simulink model "hostComms_backup_twoLoops"  (R2014b)
settings: Solver=FixedStepDiscrete  StartTime=0.0  StopTime=inf  RelTol=1e-3
InitFcn:
  | initCV;
  | 
  | fprintf('NXT init\n');
  | 
  | %try
  |  n = comms.Bt(RobotID.NXT);
  |  n.reset();
  |  n.init();
  | fprintf('NXT init done\n');
StopFcn:
  | %figure;
  | %plot(SpheroPos.signals.values(:,1), SpheroPos.signals.values(:, 2), 'kx');
  | %hold on;
  | %plot(points(:, 1), points(:, 2), 'ro');
  | %hold off
  | %axis([0 640 0 480])
  | 
  | %distEnd =  pdist([points(end, :); SpheroPos.signals.values(end, :)])
undefined symbols (not defined in the file or in its folder): angleBlue, angleOrange, curPos, curPosBlue, curPosOrange, desPos, desPosBlue, desPosOrange, Done, DoneBlue, DoneOrange, dThresh, hardcodeAngle, IsPositionTracked, IsSkeletonTracked, JointDepthIndices, JointImageIndices, JointTrackingState, JointWorldCoordinates, none, PositionDepthIndices, PositionImageIndices, PositionWorldCoordinates, posVectBlue, posVectOrange, SegmentationData, SkeletonTrackingID, Stateflow, tClose, tOpen, tSpheroStop, velocity, velocityBlue, velocityOrange, videoinput, z1Speed, z2Speed, zumoInitCentroids
undefined symbols (not defined in the file): Kd, Ki, Kp, restartspeed, RobotID, stopRadius, stopspeed
libraries: hostCommsLib x3, minionLogic x3, visiontextngfix x2, visionsinks x2, simulink x1, imaqlib x1, aerolibanimutils x1, dspvision x1
settings Model: DataDictionary=hostData.sldd  Creator=scastro  LastModifiedBy=gsalhotr

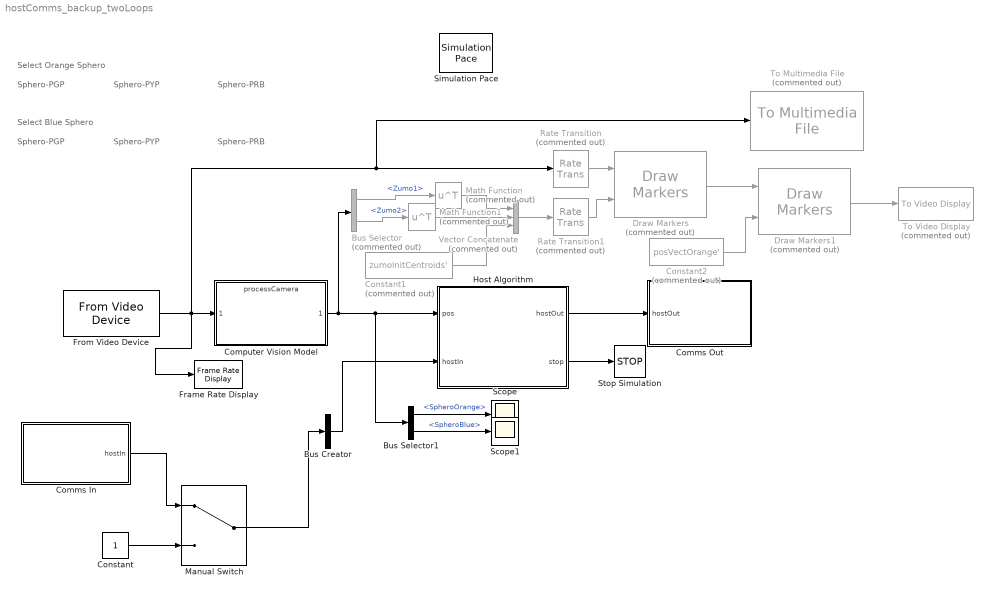
== system hostComms_backup_twoLoops ==
  note: Select Orange Sphero
  note: Sphero-PGP
  note: Sphero-PYP
  note: Sphero-PRB
  note: Select Blue Sphero
  note: Sphero-PGP
  note: Sphero-PYP
  note: Sphero-PRB
  Bus Creator : BusCreator  Inputs=1  OutDataTypeStr=Bus: CommsIn
  Bus Selector : BusSelector  Commented=on  DialogController=Simulink.DDGSource_BusSelector  OutputSignals=Zumo1,Zumo2
  Bus Selector1 : BusSelector  OutputSignals=SpheroOrange,SpheroBlue
  Comms In : Subsystem
  Comms Out : Subsystem
  Computer Vision Model : ModelReference  ModelNameDialog=processCamera  SimulationMode=Normal  ModelReferenceVersion=1.20  CopyOfModelName=processCamera  DefaultDataLogging=on
  Constant : Constant  OutDataTypeStr=uint8
  Constant1 : Constant  Commented=on  Value=zumoInitCentroids'  VectorParams1D=off
  Constant2 : Constant  Commented=on  Value=posVectOrange'
  Draw Markers : visiontextngfix/Draw Markers  Commented=on  shape=Square  size=3  fill=off  fillClrSource=Specify via dialog  display=User-specified value  intensity=200  color=[255 0 0]  opacity=0.6  viewport=Entire image  antialiasing=off  inType=Obsolete  imagePorts=One multidimensional signal  prodOutputMode=Binary point scaling  prodOutputWordLength=32  prodOutputFracLength=14  memoryMode=Specify word length  memoryWordLength=16  memoryFracLength=15  roundingMode=Floor  overflowMode=off
  Draw Markers1 : visiontextngfix/Draw Markers  Commented=on  shape=X-mark  size=3  fill=off  fillClrSource=Specify via dialog  display=User-specified value  intensity=200  color=[255 0 0]  opacity=0.6  viewport=Entire image  antialiasing=off  inType=Obsolete  imagePorts=One multidimensional signal  prodOutputMode=Binary point scaling  prodOutputWordLength=32  prodOutputFracLength=14  memoryMode=Specify word length  memoryWordLength=16  memoryFracLength=15  roundingMode=Floor  overflowMode=off
  Frame Rate Display : visionsinks/Frame Rate Display  UpdateRate=10
  From Video Device : imaqlib/From Video Device  DeviceMenu=winvideo 1 (Logitech QuickCam Pro 9000)  Device=winvideo 1 (Logitech QuickCam Pro 9000)  ObjConstructor=videoinput('winvideo', 1)  VideoFormatMenu=RGB24_640x480  VideoFormat=RGB24_640x480  VideoSource=input1  ROIPosition=[0 0 480 640]  EnableHWTrigger=off  TriggerConfiguration=none/none  SampleTime=0.2  OutputPortsMode=One multidimensional signal  DataType=single  CanDoHWTrigger=no  ReturnedColorSpace=rgb  BlockHandle=1921.0006  ROIWidth=640  ROIHeight=480  ROIColumn=0  ROIRow=0  EngXMLPath=E:\jobarchive\BR2014bd\2014_09_15_h13m58s39_job149375_pass\matlab\toolbox\imaq\imaq\private  DevXMLPath=E:\jobarchive\BR2014bd\2014_09_15_h13m58s39_job149375_pass\matlab\toolbox\imaq\supportpackages\genericvideo\adaptor\win64  EngLibPath=E:\jobarchive\BR2014bd\2014_09_15_h13m58s39_job149375_pass\matlab\toolbox\imaq\imaqblks\imaqmex\win64  ColorSpace=rgb  BayerSensorAlignment=grbg  AllMetadata=IsPositionTracked;IsSkeletonTracked;JointDepthIndices;JointImageIndices;JointTrackingState;JointWorldCoordinates;PositionDepthIndices;PositionImageIndices;PositionWorldCoordinates;SegmentationData;SkeletonTrackingID
  Host Algorithm : Stateflow chart  AncestorBlock=hostLogic/Host Algorithm  TreatAsAtomicUnit=on
  Manual Switch : ManualSwitch
  Math Function : Math  Commented=on  Operator=transpose  SaturateOnIntegerOverflow=on
  Math Function1 : Math  Commented=on  Operator=transpose  SaturateOnIntegerOverflow=on
  Rate Transition : RateTransition  Commented=on  OutPortSampleTime=1.0
  Rate Transition1 : RateTransition  Commented=on  OutPortSampleTime=1.0
  Scope : Scope
      settings: YMin=-2  YMax=0
  Scope1 : Scope
  Simulation Pace : aerolibanimutils/Simulation Pace  SimulationPace=1  SleepMode=MATLAB Thread  OutputPaceError=off  SampleTime=0.1
      settings: AttributesFormatString=%<SimulationPace> sec/sec
  Stop Simulation : Stop
  To Multimedia File : dspvision/To Multimedia File  Commented=on  outputFilename=TrialRun.mp4  streamSelection=Video only  videoCompressor=None (uncompressed)  audioCompressor=None (uncompressed)  imagePorts=One multidimensional signal  fileType=MPEG4  audioDatatype=Determine from input data type  fourcc=RGB  videoQuality=75  mj2000CompFactor=10
  To Video Display : visionsinks/To Video Display  Commented=on  inputType=Obsolete  imagePorts=One multidimensional signal  OutputDevice=On-screen video monitor  fullScreen=off  videoWindowX=710  videoWindowY=48  saveWindowSize=off  videoWindowWidth=640  videoWindowHeight=480  dataOrg=Column-major  openAtMdlStart=on  isWindowOpen=off  inputColorFormat=RGB
  Vector Concatenate : Concatenate  Commented=on  NumInputs=3  Mode=Multidimensional array
  wires:
  Bus Creator/1 -> Host Algorithm/2(hostIn)
  Host Algorithm/1(hostOut) -> Comms Out/1(hostOut)
  From Video Device/1 -> Frame Rate Display/1, Computer Vision Model/1, To Multimedia File/1, Rate Transition/1
  Host Algorithm/2(stop) -> Stop Simulation/1
  Bus Selector/1 -> Math Function/1  "<Zumo1>"
  Bus Selector/2 -> Math Function1/1  "<Zumo2>"
  Constant1/1 -> Vector Concatenate/3
  Math Function/1 -> Vector Concatenate/1
  Math Function1/1 -> Vector Concatenate/2
  Rate Transition/1 -> Draw Markers/1
  Vector Concatenate/1 -> Rate Transition1/1
  Rate Transition1/1 -> Draw Markers/2
  Computer Vision Model/1 -> Bus Selector1/1, Host Algorithm/1(pos), Bus Selector/1
  Bus Selector1/1 -> Scope/1  "<SpheroOrange>"
  Bus Selector1/2 -> Scope1/1  "<SpheroBlue>"
  Draw Markers/1 -> Draw Markers1/1
  Draw Markers1/1 -> To Video Display/1
  Constant2/1 -> Draw Markers1/2
  Comms In/1(hostIn) -> Manual Switch/1
  Constant/1 -> Manual Switch/2
  Manual Switch/1 -> Bus Creator/1

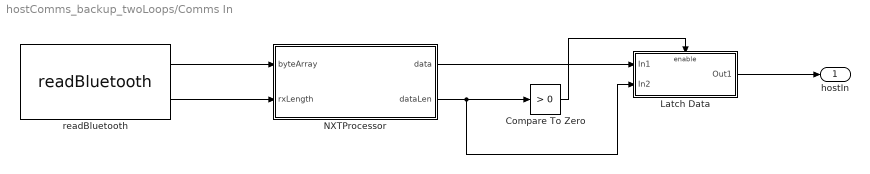
== system hostComms_backup_twoLoops/Comms In ==
  Compare To Zero : simulink/Logic and Bit Operations/Compare To Zero  relop=>  OutDataTypeStr=boolean
  Latch Data : Subsystem  TreatAsAtomicUnit=on
  NXTProcessor : MATLAB Function  TreatAsAtomicUnit=on
  readBluetooth : hostCommsLib/readBluetooth  robotId=RobotID.NXT  numBytes=4
  hostIn : Outport  OutDataTypeStr=uint8
  wires:
  Latch Data/1(Out1) -> hostIn/1
  readBluetooth/2 -> NXTProcessor/2(rxLength)
  NXTProcessor/2(dataLen) -> Latch Data/2(In2), Compare To Zero/1
  readBluetooth/1 -> NXTProcessor/1(byteArray)
  NXTProcessor/1(data) -> Latch Data/1(In1)
  Compare To Zero/1 -> Latch Data/Enable

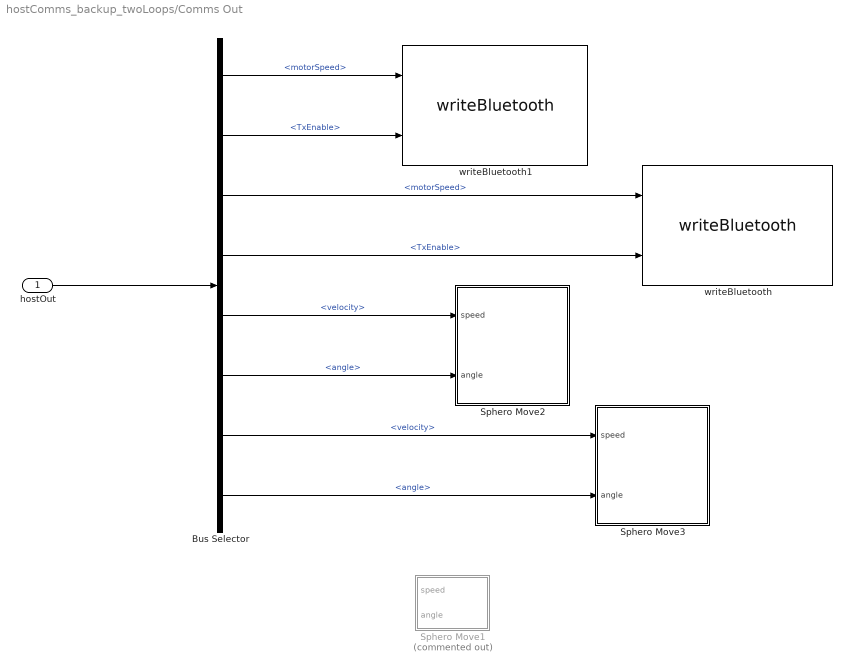
== system hostComms_backup_twoLoops/Comms Out ==
  hostOut : Inport  OutDataTypeStr=Bus: CommsOut
  Bus Selector : BusSelector  OutputSignals=Zumo1.motorSpeed,Zumo1.TxEnable,Zumo2.motorSpeed,Zumo2.TxEnable,SpheroOrange.velocity,SpheroOrange.angle,SpheroBlue.velocity,SpheroBlue.angle
  Sphero Move1 : MATLAB Function  Commented=on  TreatAsAtomicUnit=on  mask{sphero_RobotID=RobotID.SPHERO_ORANGE}
      mask prompts: sphero_RobotID "Robot"
  Sphero Move2 : MATLAB Function  TreatAsAtomicUnit=on  mask{sphero_RobotID=RobotID.SPHERO_ORANGE}
      mask prompts: sphero_RobotID "Robot"
  Sphero Move3 : MATLAB Function  TreatAsAtomicUnit=on  mask{sphero_RobotID=RobotID.SPHERO_BLUE}
      mask prompts: sphero_RobotID "Robot"
  writeBluetooth : hostCommsLib/writeBluetooth  robotId=RobotID.ZUMO_329B
  writeBluetooth1 : hostCommsLib/writeBluetooth  robotId=RobotID.ZUMO_32B0
  wires:
  hostOut/1 -> Bus Selector/1
  Bus Selector/1 -> writeBluetooth1/1  "<motorSpeed>"
  Bus Selector/2 -> writeBluetooth1/2  "<TxEnable>"
  Bus Selector/3 -> writeBluetooth/1  "<motorSpeed>"
  Bus Selector/4 -> writeBluetooth/2  "<TxEnable>"
  Bus Selector/6 -> Sphero Move2/2(angle)  "<angle>"
  Bus Selector/5 -> Sphero Move2/1(speed)  "<velocity>"
  Bus Selector/7 -> Sphero Move3/1(speed)  "<velocity>"
  Bus Selector/8 -> Sphero Move3/2(angle)  "<angle>"

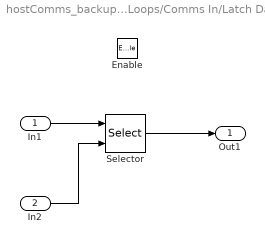
== system hostComms_backup_twoLoops/Comms In/Latch Data ==
  In1 : Inport  OutDataTypeStr=uint8
  In2 : Inport  Port=2
  Enable : EnablePort
  Selector : Selector  InputPortWidth=8  IndexOptions=Index vector (port)  Indices=[1 3]
  Out1 : Outport  OutDataTypeStr=uint8  InitialOutput=uint8(0)
  wires:
  In1/1 -> Selector/1
  Selector/1 -> Out1/1
  In2/1 -> Selector/2

== matlab function hostComms_backup_twoLoops/Comms Out/Sphero Move1 ==
  data: speed input; angle input; sphero_RobotID parameter Enum: RobotID
function fcn(speed, angle, sphero_RobotID)
%#codegen
coder.extrinsic('move_sphero_comms')

move_sphero_comms(sphero_RobotID, speed, angle);

== stateflow chart hostComms_backup_twoLoops/Host Algorithm ==
  state ZumoBot [parallel] [commented out]
  state SpheroBlue [parallel]
    settings: executionOrder=2
  state SpheroOrange [parallel]
    settings: executionOrder=3
  state Top [parallel]
    en:
    hostOut.Zumo1.motorSpeed = uint8(0);
    hostOut.Zumo1.TxEnable = 0;
    hostOut.Zumo2.motorSpeed = uint8(0);
    hostOut.Zumo2.TxEnable = 0;
    velocityOrange = 0;
    angleOrange = 0;
    velocityBlue = 0;
    angleBlue = 0;
    stop = 0;
    en,du,ex:
    % map all inputs to DSM's
    curPosOrange = pos.SpheroOrange;
    curPosBlue = pos.SpheroBlue;
    %
    % initialize des pos blue/orange for now
    %desPosOrange = [360 240]';
    %desPosBlue = [360 240]';
    settings: executionOrder=1
    state Standby
      %Wait for NXT
      %to ascend
      %mountain
    state Blink
      entry:
      spheroBlink(RobotID.SPHERO_BLUE, idx);
      spheroBlink(RobotID.SPHERO_ORANGE, idx);
      idx= idx+1;
      on every(5, tick):
      spheroBlink(RobotID.SPHERO_BLUE, idx);
      spheroBlink(RobotID.SPHERO_ORANGE, idx);
      idx= idx+1;
    state SpheroHardCodedMoveO
      en, du: MoveSphero(100, hardcodeAngle, RobotID.SPHERO_ORANGE);
    note: Workspace (sldd) Parameters
        | posVectOrange %initialized by CV
        | posVectBlue %initialized by CV
        | Kp
        | Kd
        | Ki
        | restartspeed
        | stopRadius
        | stopspeed
    state MoveOPoint1 % SpheroOrange to init point
      en:
      desPosOrange = posVectOrange(:,1);
      SpheroOrange.TurnOn();
    state MoveOPoint2 % SpheroOrange to gate
      en:
      desPosOrange = posVectOrange(:,2);
      SpheroOrange.TurnOn();
    state SpheroHardCodedMoveB
      en, du: MoveSphero(100, hardcodeAngle, RobotID.SPHERO_BLUE);
    state MoveBPoint1 % SpheroBlue to init point
      en:
      desPosBlue = posVectBlue(:,1);
      SpheroBlue.TurnOn();
    state tf = zumoClose(initPos,curPos,dTh) [function]
      (default) -> (junction 130) : {tf = norm(curPos.Zumo1 - initPos(:,1)) <= dTh;}
    state Blink1
      entry:
      idx = 1;
      spheroBlink(RobotID.SPHERO_ORANGE, idx);
      idx= idx+1;
      on every(5, tick):
      spheroBlink(RobotID.SPHERO_ORANGE, idx);
      idx= idx+1;
    state State2 % Zumo open gate
      en:
      hostOut.Zumo1.motorSpeed = uint8(z1Speed);
      hostOut.Zumo1.TxEnable = 1;
      hostOut.Zumo2.motorSpeed = uint8(z2Speed);
      hostOut.Zumo2.TxEnable = 1;
      ex:
      hostOut.Zumo1.motorSpeed = uint8(0);
      hostOut.Zumo2.motorSpeed = uint8(0);
    state State3 % SpheroOrange Move to center
      en:
      desPosOrange = posVectOrange(:,3);
      SpheroOrange.TurnOn()
    state State4 % Zumo begin close gate
      en:
      hostOut.Zumo1.motorSpeed = uint8(z1Speed);
      hostOut.Zumo2.motorSpeed = uint8(z2Speed);
    state State5 % Zumo stop
      en:
      hostOut.Zumo1.motorSpeed = uint8(0);
      hostOut.Zumo2.motorSpeed = uint8(0);
    state State6 % SpheroBlue to gate
      en:
      desPosBlue = posVectBlue(:,2);
      SpheroBlue.TurnOn();
    state Blink2
      entry:
      idx = 1;
      spheroBlink(RobotID.SPHERO_BLUE, idx);
      idx= idx+1;
      on every(5, tick):
      spheroBlink(RobotID.SPHERO_BLUE, idx);
      idx= idx+1;
    state State7 % Zumo open gate
      en:
      hostOut.Zumo1.motorSpeed = uint8(z1Speed);
      hostOut.Zumo1.TxEnable = 1;
      hostOut.Zumo2.motorSpeed = uint8(z2Speed);
      hostOut.Zumo2.TxEnable = 1;
      ex:
      hostOut.Zumo1.motorSpeed = uint8(0);
      hostOut.Zumo2.motorSpeed = uint8(0);
    state State8 % SpheroBlue Move to center
      en:
      desPosBlue = posVectBlue(:,3);
      SpheroBlue.TurnOn()
    state State9 % Zumo begin close gate
      en:
      hostOut.Zumo1.motorSpeed = uint8(z1Speed);
      hostOut.Zumo2.motorSpeed = uint8(z2Speed);
    state State10 % Zumo stop
      en:
      hostOut.Zumo1.motorSpeed = uint8(0);
      hostOut.Zumo2.motorSpeed = uint8(0);
    state State11 %Stop model
      en: stop = 1;
    (default) -> Standby
    Standby -> Blink : [hostIn.NXT == 1 || hostIn.NXT == 99 || after(90,sec)]{idx = 1;}
    Blink -> SpheroHardCodedMoveO : [idx>5]{spheroBlink(RobotID.SPHERO_BLUE, 8);
        | 		spheroBlink(RobotID.SPHERO_ORANGE, 8);}
    SpheroHardCodedMoveO -> MoveOPoint1 % SpheroOrange to init point : [all(curPosOrange>0)]
    MoveOPoint1 % SpheroOrange to init point -> MoveOPoint2 % SpheroOrange to gate [order 1] : [DoneOrange]
    MoveOPoint1 % SpheroOrange to init point -> MoveOPoint2 % SpheroOrange to gate [order 2] : [after(tSpheroStop, sec)]{SpheroOrange.TurnOff;}
        | %condition when sphero is done moving?
    MoveOPoint2 % SpheroOrange to gate -> SpheroHardCodedMoveB [order 2] : [DoneOrange]
    MoveOPoint2 % SpheroOrange to gate -> SpheroHardCodedMoveB [order 1] : [after(tSpheroStop, sec)]{SpheroOrange.TurnOff;}
        | %condition when sphero is done moving?
    SpheroHardCodedMoveB -> MoveBPoint1 % SpheroBlue to init point : [all(curPosBlue>0)]
    MoveBPoint1 % SpheroBlue to init point -> Blink1 [order 1] : [DoneBlue]
    MoveBPoint1 % SpheroBlue to init point -> Blink1 [order 2] : [after(tSpheroStop, sec)]{SpheroBlue.TurnOff;}
        | %condition when sphero is done moving?
    Blink1 -> State2 % Zumo open gate : [idx>7]{spheroBlink(RobotID.SPHERO_ORANGE, 8)}
    State2 % Zumo open gate -> State3 % SpheroOrange Move to center : after(tOpen,sec)
    State3 % SpheroOrange Move to center -> State4 % Zumo begin close gate [order 2] : [DoneOrange]
    State3 % SpheroOrange Move to center -> State4 % Zumo begin close gate [order 1] : [after(tSpheroStop, sec)]{SpheroOrange.TurnOff;}
        | %condition when sphero is done moving?
    State4 % Zumo begin close gate -> State5 % Zumo stop : [after(tClose,sec)]
    State5 % Zumo stop -> State6 % SpheroBlue to gate
    State6 % SpheroBlue to gate -> Blink2 [order 2] : [DoneBlue]
    State6 % SpheroBlue to gate -> Blink2 [order 1] : [after(tSpheroStop, sec)]{SpheroBlue.TurnOff;}
        | %condition when sphero is done moving?
    Blink2 -> State7 % Zumo open gate : [idx>7]{spheroBlink(RobotID.SPHERO_BLUE, 8)}
    State7 % Zumo open gate -> State8 % SpheroBlue Move to center : after(tOpen,sec)
    State8 % SpheroBlue Move to center -> State9 % Zumo begin close gate [order 1] : [DoneBlue]
    State8 % SpheroBlue Move to center -> State9 % Zumo begin close gate [order 2] : [after(tSpheroStop, sec)]{SpheroBlue.TurnOff;}
        | %condition when sphero is done moving?
    State9 % Zumo begin close gate -> State10 % Zumo stop : [after(tClose,sec)]
    State10 % Zumo stop -> State11 %Stop model
  state Exit [parallel]
    en,du,ex:
    % Initializing here until filled into algorithm
    % Write DSM's to outputs
    hostOut.SpheroOrange.velocity = velocityOrange;
    hostOut.SpheroOrange.angle = angleOrange;
    hostOut.SpheroBlue.velocity = velocityBlue;
    hostOut.SpheroBlue.angle = angleBlue;
    settings: executionOrder=4
  data: robot function_input; index function_input; initPos function_input; curPos function_input; dTh function_input; tf function_output; speed function_input; angle function_input; sphero_RobotID function_input; pos input Bus: PositionBus size=1; hostIn input Bus: CommsIn size=1; hostOut output Bus: CommsOut size=1; desPosBlue local double size=2; desPosOrange local double size=2; curPosBlue local double size=2; curPosOrange local double size=2; velocityOrange local double size=1; angleOrange local double size=1; velocityBlue local double size=1; angleBlue local double size=1; posVectBlue parameter double; posVectOrange parameter double; DoneOrange local boolean size=1; DoneBlue local boolean size=1; zumoInitCentroids parameter; dThresh parameter double =10; tClose parameter double =5; stop output; tSpheroStop parameter; tOpen parameter; idx local; hardcodeAngle parameter; z1Speed parameter; z2Speed parameter
  function spheroBlink(robot, index):
    | function spheroBlink(robot, index)
    |  
    | coder.extrinsic('spheroBlinking');
    | 
    | spheroBlinking(robot, index);
  function MoveSphero(speed, angle, sphero_RobotID):
    | function MoveSphero(speed, angle, sphero_RobotID)
    | %#codegen
    | coder.extrinsic('move_sphero_comms')
    | 
    | move_sphero_comms(sphero_RobotID, speed, angle);

== matlab function hostComms_backup_twoLoops/Comms In/NXTProcessor ==
  data: data output uint8; dataLen output; byteArray input uint8; rxLength input double; NXTBufferSize parameter
function [data,dataLen] = nxtProcessor(byteArray,rxLength, NXTBufferSize)
%#codegen

persistent NXT;

if(isempty(NXT))
    bufferLen = uint8(NXTBufferSize);
    NXT = comms.RawNXTDataProcessor(bufferLen);
end

[data,dataLen] = NXT.process(byteArray,uint8(rxLength));

end

== matlab function hostComms_backup_twoLoops/Comms Out/Sphero Move3 ==
  data: speed input; angle input; sphero_RobotID parameter Enum: RobotID
function fcn(speed, angle, sphero_RobotID)
%#codegen
coder.extrinsic('move_sphero_comms')

move_sphero_comms(sphero_RobotID, speed, angle);

== matlab function hostComms_backup_twoLoops/Comms Out/Sphero Move2 ==
  data: speed input; angle input; sphero_RobotID parameter Enum: RobotID
function fcn(speed, angle, sphero_RobotID)
%#codegen
coder.extrinsic('move_sphero_comms')

move_sphero_comms(sphero_RobotID, speed, angle);
